simulink model "Week_5_Time_delay"  (R2016a)
settings: Solver=FixedStepAuto  StartTime=0.0  StopTime=10.0  FixedStep=0.001  RelTol=1e-3
PreLoadFcn:
  | a=1;
  | sim(Week_5_Time_delay.slx');
  | if a==1
  |   sim('PID_Kim.slx')
  | end
values from neighbouring files (symbols this model uses):
  D = 0.53908    [Tut_Week_5.m]
  I = 25.0289    [Tut_Week_5.m]
  Kp = 100    [Tut_Week_5.m]
  Ks = 0.1    [Tut_Week_5.m]
  L = 0.1    [Tut_Week_5.m]
  N = 6.4951    [Tut_Week_5.m]    (also in Week_8_Final.m = 20)
  P = 15.376    [Tut_Week_5.m]
  T = 1    [Tut_Week_5.m]
libraries: simulink x1
settings Model: Creator=김태욱  LastModifiedBy=김태욱

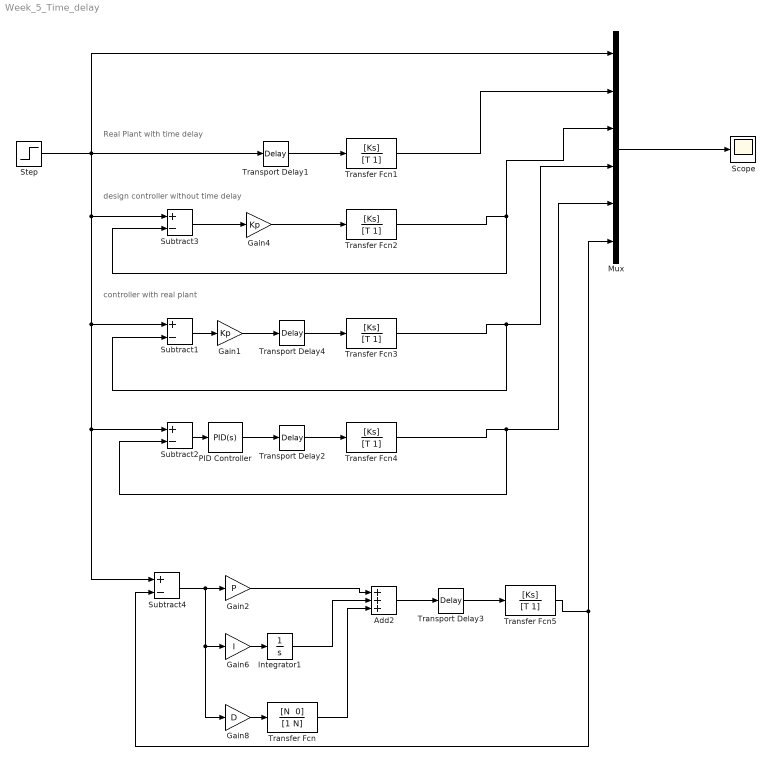
== system Week_5_Time_delay ==
  note: controller with real plant
  note: design controller without time delay
  note: Real Plant with time delay
  Add2 : Sum  Inputs=+++
  Gain1 : Gain  Gain=Kp
  Gain2 : Gain  Gain=P
  Gain4 : Gain  Gain=Kp
  Gain6 : Gain  Gain=I
  Gain8 : Gain  Gain=D
  Integrator1 : Integrator
  Mux : Mux  Inputs=6
  PID Controller : simulink/Continuous/PID Controller  Controller=PID  TimeDomain=Continuous-time  SampleTime=-1  IntegratorMethod=Forward Euler  FilterMethod=Forward Euler  Form=Parallel  UseFilter=on  ControllerParametersSource=internal  P=1  I=1  D=0  N=100  InitialConditionSource=internal  InitialConditionForIntegrator=0  InitialConditionForFilter=0  ExternalReset=none  LimitOutput=off  UpperSaturationLimit=inf  LowerSaturationLimit=-inf  LinearizeAsGain=on  AntiWindupMode=none  Kb=1  TrackingMode=off  Kt=1  PParamMin=[]  PParamMax=[]  IParamMin=[]  IParamMax=[]  DParamMin=[]  DParamMax=[]  NParamMin=[]  NParamMax=[]  KbParamMin=[]  KbParamMax=[]  KtParamMin=[]  KtParamMax=[]  POutMin=[]  POutMax=[]  IOutMin=[]  IOutMax=[]  DOutMin=[]  DOutMax=[]  NOutMin=[]  NOutMax=[]  KbOutMin=[]  KbOutMax=[]  KtOutMin=[]  KtOutMax=[]  IntegratorOutMin=[]  IntegratorOutMax=[]  FilterOutMin=[]  FilterOutMax=[]  SumOutMin=[]  SumOutMax=[]  SumI1OutMin=[]  SumI1OutMax=[]  SumI2OutMin=[]  SumI2OutMax=[]  SumI3OutMin=[]  SumI3OutMax=[]  SumDOutMin=[]  SumDOutMax=[]  SaturationOutMin=[]  SaturationOutMax=[]  IntegratorContinuousStateAttributes=''  IntegratorStateMustResolveToSignalObject=off  IntegratorRTWStateStorageClass=Auto  FilterContinuousStateAttributes=''  FilterStateMustResolveToSignalObject=off  FilterRTWStateStorageClass=Auto  DifferentiatorICPrevScaledInput=0  DifferentiatorOutMin=[]  DifferentiatorOutMax=[]
  Scope : Scope
  Step : Step  SampleTime=0
  Subtract{1..4} (4 alike) : Sum  Inputs=+-
  Transfer Fcn : TransferFcn  Numerator="[N  0]"  Denominator=[1 N]
  Transfer Fcn{1..5} (5 alike) : TransferFcn  Numerator=[Ks]  Denominator=[T 1]
  Transport Delay{1..4} (4 alike) : TransportDelay  DelayTime=L
  wires:
  Gain4/1 -> Transfer Fcn2/1
  Transfer Fcn2/1 -> Subtract3/2, Mux/3
  Subtract3/1 -> Gain4/1
  Transport Delay4/1 -> Transfer Fcn3/1
  Transfer Fcn3/1 -> Mux/4, Subtract1/2
  Subtract1/1 -> Gain1/1
  Gain1/1 -> Transport Delay4/1
  Transport Delay1/1 -> Transfer Fcn1/1
  Transport Delay2/1 -> Transfer Fcn4/1
  Transfer Fcn4/1 -> Mux/5, Subtract2/2
  Subtract2/1 -> PID Controller/1
  PID Controller/1 -> Transport Delay2/1
  Step/1 -> Transport Delay1/1, Subtract4/1, Subtract2/1, Subtract1/1, Subtract3/1, Mux/1
  Gain2/1 -> Add2/1
  Add2/1 -> Transport Delay3/1
  Transfer Fcn5/1 -> Mux/6, Subtract4/2
  Gain6/1 -> Integrator1/1
  Integrator1/1 -> Add2/2
  Subtract4/1 -> Gain2/1, Gain8/1, Gain6/1
  Gain8/1 -> Transfer Fcn/1
  Transfer Fcn/1 -> Add2/3
  Mux/1 -> Scope/1
  Transport Delay3/1 -> Transfer Fcn5/1
  Transfer Fcn1/1 -> Mux/2
